simulink model "validate_density_mdl"  (Simulink 7.6)
settings: Solver=FixedStepDiscrete  StartTime=0.0  StopTime=1  FixedStep=1  RelTol=1e-3
values from neighbouring files (symbols this model uses):
  fmix = mix(n)    [verification_density.m]    (also in verification_fluidproperty.m; verification_heat_capacity.m; verification_kinematic_viscosity.m; verification_thermal_conductivity.m)
  press = p(m)    [verification_density.m]    (also in verification_fluidproperty.m; verification_heat_capacity.m; verification_kinematic_viscosity.m; verification_thermal_conductivity.m)
undefined symbols (not defined in the file or in its folder): fluid
libraries: carnot x1
settings Model: Creator=drhf  LastModifiedBy=drhf
settings DataIOCC: SaveTime=off  ReturnWorkspaceOutputs=on  OutputSaveName=rho2

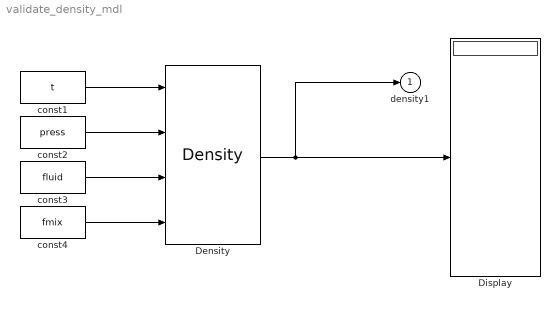
== system validate_density_mdl ==
  Density : carnot/Basic/Material_Properties/Density  SystemSampleTime=-1
  Display : Display
  const1 : Constant  Value=t
  const2 : Constant  Value=press
  const3 : Constant  Value=fluid
  const4 : Constant  Value=fmix
  density1 : Outport  InitialOutput=0
  wires:
  const2/1 -> Density/2
  const3/1 -> Density/3
  const4/1 -> Density/4
  const1/1 -> Density/1
  Density/1 -> Display/1, density1/1
